simulink model "Modello_Maglev_finale_LQR"  (R2022b)
settings: Solver=FixedStepAuto  StartTime=0.0  StopTime=10  FixedStep=dt  RelTol=1e-3
undefined symbols (not defined in the file): BallDiam, BallMass, Drag, dt, EMsDist, g, K_LQR_int, m, Res, ueq, x_d
libraries: simulink x1
settings Model: Creator=User  LastModifiedBy=anton
settings DebuggingCC: UnconnectedInputMsg=warning  UnconnectedOutputMsg=warning  UnconnectedLineMsg=warning
settings ModelReferenceCC: EnableRefExpFcnMdlSchedulingChecks=on
settings RTWCC: DLArmComputeVersion=19.05

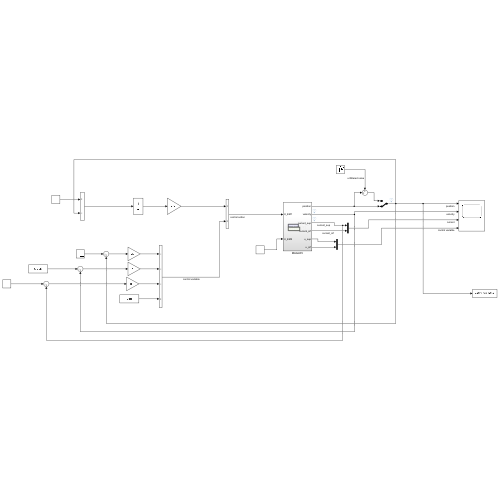
[thumbnail: Simulink's stored preview of the top-level diagram]
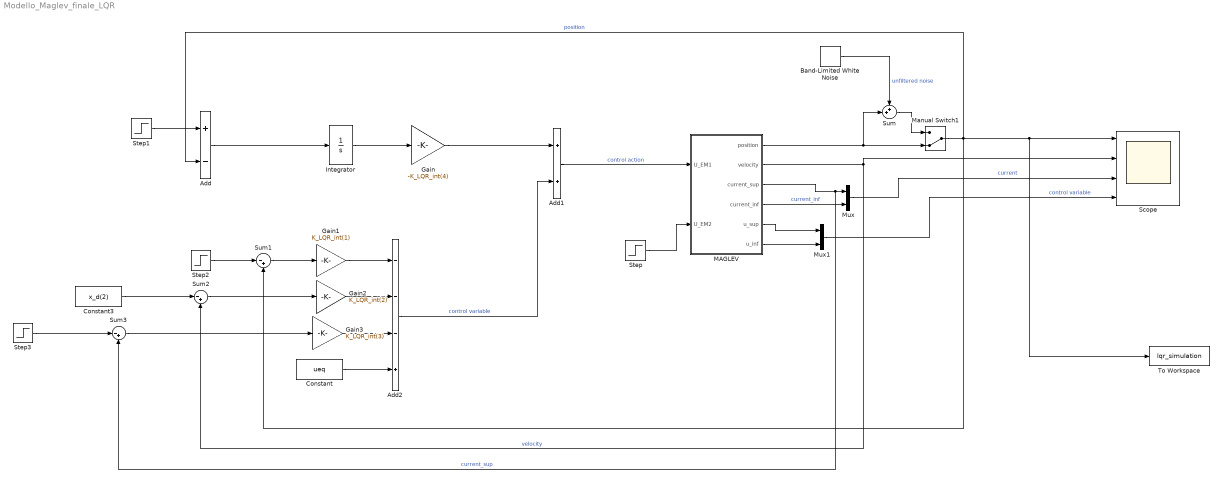
== system Modello_Maglev_finale_LQR ==
  Add : Sum  Inputs=+-
  Add1 : Sum
  Add2 : Sum  Inputs=---+
  Band-Limited White Noise : simulink/Sources/Band-Limited White Noise  Cov=[0.000000000003]  Ts=dt  seed=[23341]
  Constant : Constant  Value=ueq
  Constant3 : Constant  Value=x_d(2)
  Gain : Gain  Gain=-K_LQR_int(4)
  Gain1 : Gain  Gain=K_LQR_int(1)
  Gain2 : Gain  Gain=K_LQR_int(2)
  Gain3 : Gain  Gain=K_LQR_int(3)
  Integrator : Integrator
  MAGLEV : Subsystem
  Manual Switch1 : ManualSwitch  CurrentSetting=0
  Mux : Mux  Inputs=2
  Mux1 : Mux  Inputs=2
  Scope : Scope  NumInputPorts=4
  Step : Step  Time=0  After=0  SampleTime=0
  Step1 : Step  Time=0.18  Before=0.0143  After=0.01  SampleTime=0
  Step2 : Step  Time=0.18  Before=0.0143  After=0.01  SampleTime=0
  Step3 : Step  Time=0.18  After=x_d(3)  SampleTime=0
  Sum : Sum  Inputs=++|
  Sum1 : Sum  Inputs=|-+
  Sum2 : Sum  Inputs=|-+
  Sum3 : Sum  Inputs=|-+
  To Workspace : ToWorkspace  VariableName=lqr_simulation  SaveFormat=Structure With Time  SampleTime=-1
  wires:
  Step/1 -> MAGLEV/2(U_EM2)
  MAGLEV/4(current_inf) -> Mux/2  "current_inf"
  Mux/1 -> Scope/3  "current"
  MAGLEV/5(u_sup) -> Mux1/1
  MAGLEV/6(u_inf) -> Mux1/2
  Mux1/1 -> Scope/4  "control variable"
  MAGLEV/1(position) -> Manual Switch1/2, Sum/2
  Band-Limited White Noise/1 -> Sum/1  "unfiltered noise"
  Sum/1 -> Manual Switch1/1
  Add1/1 -> MAGLEV/1(U_EM1)  "control action"
  Integrator/1 -> Gain/1
  Step1/1 -> Add/1
  Add/1 -> Integrator/1
  Gain/1 -> Add1/1
  Step2/1 -> Sum1/1
  Gain1/1 -> Add2/1
  Step3/1 -> Sum3/1
  Constant3/1 -> Sum2/1
  Sum2/1 -> Gain2/1
  Sum3/1 -> Gain3/1
  Gain3/1 -> Add2/3
  Gain2/1 -> Add2/2
  Constant/1 -> Add2/4
  Manual Switch1/1 -> Sum1/2, To Workspace/1, Scope/1, Add/2  "position"
  MAGLEV/3(current_sup) -> Mux/1, Sum3/2  "current_sup"
  Add2/1 -> Add1/2  "control variable"
  Sum1/1 -> Gain1/1
  MAGLEV/2(velocity) -> Sum2/2, Scope/2  "velocity"

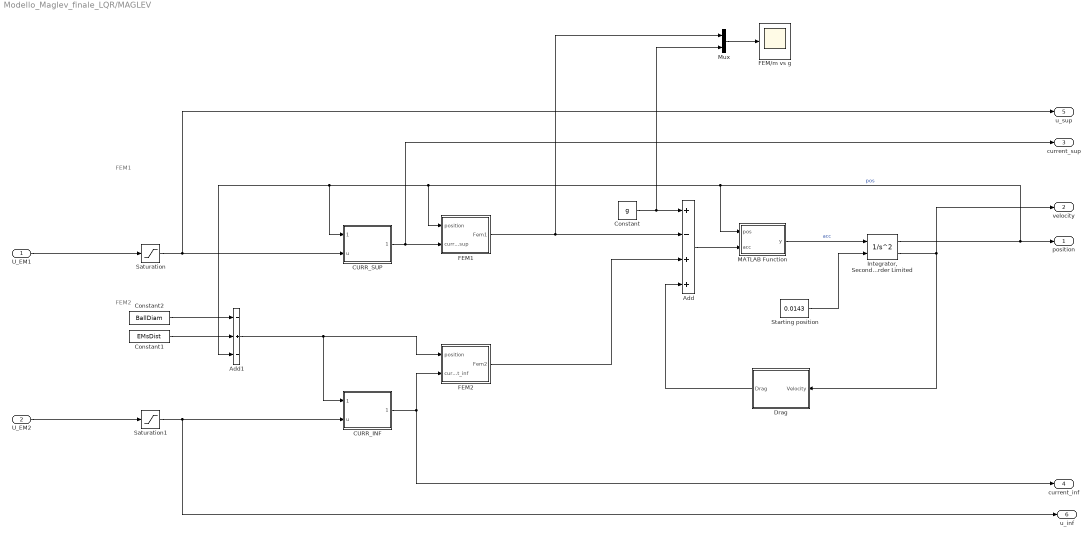
== system Modello_Maglev_finale_LQR/MAGLEV ==
  note: FEM1
  note: FEM2
  U_EM1 : Inport
  U_EM2 : Inport  Port=2
  Add : Sum  Inputs=+-++
  Add1 : Sum  Inputs=-+-
  CURR_INF : Subsystem
  CURR_SUP : Subsystem
  Constant : Constant  Value=g
  Constant1 : Constant  Value=EMsDist
  Constant2 : Constant  Value=BallDiam
  Drag : Subsystem
  FEM/m vs g : Scope
  FEM1 : Subsystem
  FEM2 : Subsystem
  "Integrator, Second-Order Limited" : SecondOrderIntegrator  ICSourceX=external  LimitX=on  UpperLimitX=0.0143  LowerLimitX=0  LimitDXDT=on
  MATLAB Function : MATLAB Function  TreatAsAtomicUnit=on
  Mux : Mux  Inputs=2
  Saturation : Saturate  UpperLimit=1  LowerLimit=0
  Saturation1 : Saturate  UpperLimit=1  LowerLimit=0
  Starting position : Constant  Value=0.0143
  position : Outport
  velocity : Outport  Port=2
  current_sup : Outport  Port=3
  current_inf : Outport  Port=4
  u_sup : Outport  Port=5
  u_inf : Outport  Port=6
  wires:
  U_EM1/1 -> Saturation/1
  "Integrator, Second-Order Limited"/1 -> position/1, MATLAB Function/1(pos), FEM1/1(position), CURR_SUP/1(position), Add1/3  "pos"
  U_EM2/1 -> Saturation1/1
  Constant/1 -> Mux/2, Add/1
  CURR_INF/1(current_inf) -> FEM2/2(current_inf), current_inf/1
  Add1/1 -> CURR_INF/1(position), FEM2/1(position)
  Constant1/1 -> Add1/2
  Constant2/1 -> Add1/1
  CURR_SUP/1(current_sup) -> current_sup/1, FEM1/2(current_sup)
  Saturation1/1 -> CURR_INF/2(u), u_inf/1
  FEM1/1(Fem1) -> Add/2, Mux/1
  Saturation/1 -> u_sup/1, CURR_SUP/2(u)
  FEM2/1(Fem2) -> Add/3
  Mux/1 -> FEM/m vs g/1
  Starting position/1 -> "Integrator, Second-Order Limited"/2
  MATLAB Function/1(y) -> "Integrator, Second-Order Limited"/1  "acc"
  Add/1 -> MATLAB Function/2(acc)
  "Integrator, Second-Order Limited"/2 -> Drag/1(Velocity), velocity/1
  Drag/1(Drag) -> Add/4

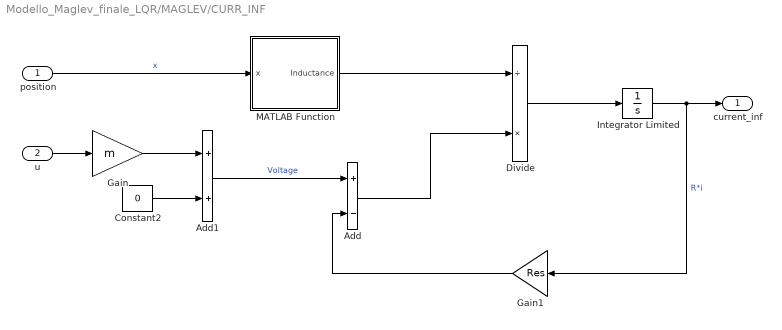
== system Modello_Maglev_finale_LQR/MAGLEV/CURR_INF ==
  position : Inport
  u : Inport  Port=2
  Add : Sum  Inputs=+-
  Add1 : Sum
  Constant2 : Constant  Value=0
  Divide : Product  Inputs=/*
  Gain : Gain  Gain=m
  Gain1 : Gain  Gain=Res
  Integrator Limited : Integrator  UpperSaturationLimit=1  LowerSaturationLimit=0
  MATLAB Function : MATLAB Function  TreatAsAtomicUnit=on
  current_inf : Outport
  wires:
  Add1/1 -> Add/1  "Voltage"
  Integrator Limited/1 -> Gain1/1, current_inf/1  "R*i"
  position/1 -> MATLAB Function/1(x)  "x"
  Add/1 -> Divide/2
  Divide/1 -> Integrator Limited/1
  MATLAB Function/1(Inductance) -> Divide/1
  Gain/1 -> Add1/1
  u/1 -> Gain/1
  Constant2/1 -> Add1/2
  Gain1/1 -> Add/2

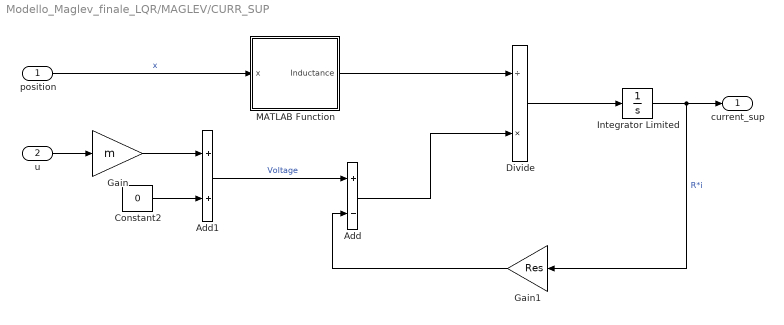
== system Modello_Maglev_finale_LQR/MAGLEV/CURR_SUP ==
  position : Inport
  u : Inport  Port=2
  Add : Sum  Inputs=+-
  Add1 : Sum
  Constant2 : Constant  Value=0
  Divide : Product  Inputs=/*
  Gain : Gain  Gain=m
  Gain1 : Gain  Gain=Res
  Integrator Limited : Integrator  UpperSaturationLimit=1  LowerSaturationLimit=0
  MATLAB Function : MATLAB Function  TreatAsAtomicUnit=on
  current_sup : Outport
  wires:
  Add1/1 -> Add/1  "Voltage"
  Integrator Limited/1 -> Gain1/1, current_sup/1  "R*i"
  position/1 -> MATLAB Function/1(x)  "x"
  Add/1 -> Divide/2
  Divide/1 -> Integrator Limited/1
  MATLAB Function/1(Inductance) -> Divide/1
  Gain/1 -> Add1/1
  u/1 -> Gain/1
  Constant2/1 -> Add1/2
  Gain1/1 -> Add/2

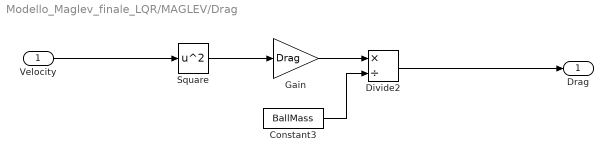
== system Modello_Maglev_finale_LQR/MAGLEV/Drag ==
  Velocity : Inport
  Constant3 : Constant  Value=BallMass
  Divide2 : Product  Inputs=*/
  Gain : Gain  Gain=Drag
  Square : Math  Operator=square
  Drag : Outport
  wires:
  Square/1 -> Gain/1
  Velocity/1 -> Square/1
  Constant3/1 -> Divide2/2
  Gain/1 -> Divide2/1
  Divide2/1 -> Drag/1

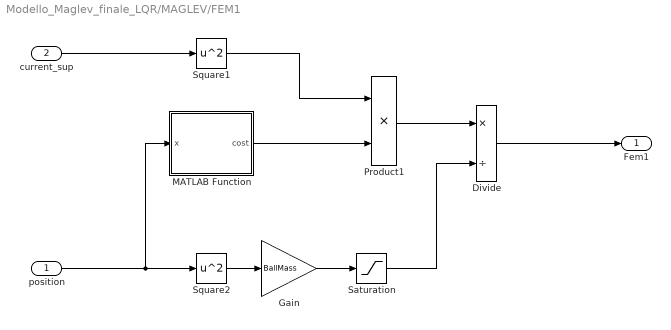
== system Modello_Maglev_finale_LQR/MAGLEV/FEM1 ==
  position : Inport
  current_sup : Inport  Port=2
  Divide : Product  Inputs=*/
  Gain : Gain  Gain=BallMass
  MATLAB Function : MATLAB Function  TreatAsAtomicUnit=on
  Product1 : Product
  Saturation : Saturate  UpperLimit=40  LowerLimit=0.00000001
  Square1 : Math  Operator=square
  Square2 : Math  Operator=square
  Fem1 : Outport
  wires:
  position/1 -> MATLAB Function/1(x), Square2/1
  current_sup/1 -> Square1/1
  Product1/1 -> Divide/1
  Square2/1 -> Gain/1
  Divide/1 -> Fem1/1
  MATLAB Function/1(cost) -> Product1/2
  Square1/1 -> Product1/1
  Saturation/1 -> Divide/2
  Gain/1 -> Saturation/1

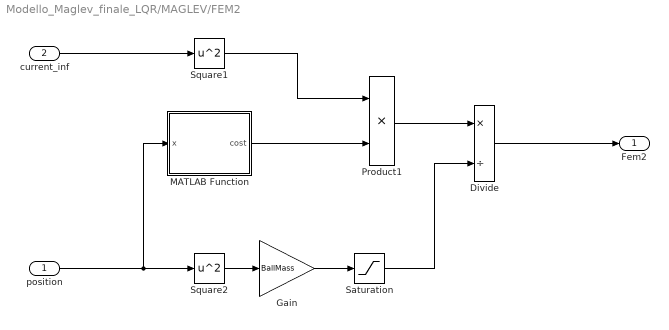
== system Modello_Maglev_finale_LQR/MAGLEV/FEM2 ==
  position : Inport
  current_inf : Inport  Port=2
  Divide : Product  Inputs=*/
  Gain : Gain  Gain=BallMass
  MATLAB Function : MATLAB Function  TreatAsAtomicUnit=on
  Product1 : Product
  Saturation : Saturate  UpperLimit=40  LowerLimit=0.00000001
  Square1 : Math  Operator=square
  Square2 : Math  Operator=square
  Fem2 : Outport
  wires:
  position/1 -> MATLAB Function/1(x), Square2/1
  current_inf/1 -> Square1/1
  Product1/1 -> Divide/1
  Square2/1 -> Gain/1
  Divide/1 -> Fem2/1
  MATLAB Function/1(cost) -> Product1/2
  Square1/1 -> Product1/1
  Saturation/1 -> Divide/2
  Gain/1 -> Saturation/1

== matlab function Modello_Maglev_finale_LQR/MAGLEV/FEM2/MATLAB Function ==
  data: x input; cost output
function cost=kem2(x)

xd = 0.0360;
Kem_2 = 1.0e-04*[0.7393 0.7614 0.7616 0.7487 0.7694 0.7763 0.7481 0.7713 0.7755 0.7761 0.7683];
pos_2 = xd - [0.0176 0.0166 0.016 0.01529 0.01429 0.0130 0.0125 0.01 0.0084 0.006 0.0026];

if x<=pos_2(1)
    cost=Kem_2(1);
elseif x<=pos_2(end) && x>=pos_2(1)
    cost=interp1(pos_2,Kem_2,x);
else 
    cost=Kem_2(end)*x/pos_2(end);
end

== matlab function Modello_Maglev_finale_LQR/MAGLEV/CURR_SUP/MATLAB Function ==
  data: x input; Inductance output
function Inductance=Inductance(x)

L = [0.1120    0.1200    0.1200    0.1240    0.1320    0.1400    0.1440];
pos_L = [0.0177    0.0165    0.0126    0.0076    0.0044    0.0019    0.0000];

if x>=pos_L(1)
    Inductance=L(1);
elseif x>=pos_L(end) && x<=pos_L(1)
    Inductance=interp1(pos_L,L,x);
else 
    Inductance=L(end);
end

== matlab function Modello_Maglev_finale_LQR/MAGLEV/FEM1/MATLAB Function ==
  data: x input; cost output
function cost=kem1(x)
kem_1=[6.72059206644115e-05	6.92145376989519e-05	6.92332150285897e-05	6.80659146785482e-05	6.99479714473845e-05	7.05722629122651e-05	6.80128124860478e-05	7.01221702001213e-05	7.05016878442255e-05	7.05515419323440e-05	6.98455307642310e-05	7.13055533313152e-05	6.96274521174565e-05	6.90147402074580e-05	6.99419931300404e-05	6.95805738707539e-05	6.93269258852514e-05	6.90843621353604e-05	7.00006512636940e-05	6.91149414076029e-05	6.97519014539535e-05	6.83573053782350e-05	6.89933518537361e-05	6.79953062557338e-05	6.77206336827605e-05	6.82595333358458e-05	6.6494e-05	6.41548968339966e-05	6.08172215535155e-05	6.05299131311581e-05	6.01818568879911e-05	5.87123846492744e-05	5.77159494392489e-05	5.52986546480238e-05	5.22809928128838e-05	4.60062308129917e-05	4.12885327629886e-05	3.57707157204477e-05	2.88156521526937e-05	2.23928764595895e-05	1.69237291476886e-05];
pos_1=[0.0194279333333333	0.0190477333333333	0.0188606000000000	0.0181366333333333	0.0178862666666667	0.0176649333333333	0.0172163000000000	0.0169433666666667	0.0166807000000000	0.0164495000000000	0.0160222000000000	0.0153453666666667	0.0148285333333333	0.0144294333333333	0.0141447000000000	0.0138273666666667	0.0133592000000000	0.0130921666666667	0.0128335333333333	0.0124948500000000	0.0121420000000000	0.0118023333333333	0.0114197500000000	0.0110494800000000	0.0106465400000000	0.0103677000000000	0.0100000000000000	0.00959026666666667	0.00925280000000000	0.00890150000000000	0.00854740000000000	0.00817620000000000	0.00779310000000000	0.00711953333333333	0.00644370000000000	0.00575746666666667	0.00497293333333333	0.00423913333333333	0.00351336666666667	0.00277350000000000	0.00202256666666667];
if x>=pos_1(1)
    cost=kem_1(1);
elseif x>=pos_1(end) && x<=pos_1(1)
    cost=interp1(pos_1,kem_1,x);
else 
    cost=kem_1(end)*x/pos_1(end);
end

== matlab function Modello_Maglev_finale_LQR/MAGLEV/CURR_INF/MATLAB Function ==
  data: x input; Inductance output
function Inductance=Inductance(x)

L2 = [0.1200 0.1200 0.1200 0.1200 0.1200 0.1200 0.1200 0.1200 0.1200];
pos_L2 = [0.0194 0.0214 0.0221 0.0229 0.0238 0.0248 0.0266 0.0335 0.0351];

if x<=pos_L2(1)
    Inductance=L2(1);
elseif x<=pos_L2(end) && x>=pos_L2(1)
    Inductance=interp1(pos_L2,L2,x);
else 
    Inductance=L2(end);
end

== matlab function Modello_Maglev_finale_LQR/MAGLEV/MATLAB Function ==
  data: pos input; y output; acc input
function y = fcn(pos,acc)
if (pos == 0.0185 && acc > 0) || (pos == 0 && acc<0)
    y = 0;
else
    y = acc;
end
